simulink library "BrickPi"  (R2018b)
settings: Solver=VariableStepAuto  StartTime=0.0  StopTime=10.0  RelTol=1e-3
libraries: raspberrypilib x50, hdlsllib x27, xpcutilitieslib x18, $bdroot x1
(part 4 of 4)

== system BrickPi/Motor_Encoder/Get Encoder Value/Switch Case Action Subsystem/Subsystem/Motor_Offset ==
  note: Set offset value
  Offset : Inport  OutDataTypeStr=int32
  MotorPort : Inport  Port=2  OutDataTypeStr=uint8
  "Address " : Constant  OutDataTypeStr=uint8
  Bit Shift : hdlsllib/Logic and Bit Operations/Bit Shift  mode=Shift Right Logical  N=24
      settings: SourceProductName=HDL Coder  SourceProductBaseCode=HD
  Bit Shift1 : hdlsllib/Logic and Bit Operations/Bit Shift  mode=Shift Right Logical  N=16
      settings: SourceProductName=HDL Coder  SourceProductBaseCode=HD
  Bit Shift2 : hdlsllib/Logic and Bit Operations/Bit Shift  mode=Shift Right Logical  N=8
      settings: SourceProductName=HDL Coder  SourceProductBaseCode=HD
  Constant2 : Constant  OutDataTypeStr=uint8
  Constant3 : Constant  OutDataTypeStr=uint8
  Data Type Conversion{,1..3} (4 alike) : DataTypeConversion  OutDataTypeStr=uint8
  Mux2 : Mux  Inputs=7
  SPI Master Transfer2 : raspberrypilib/SPI Master Transfer  Priority=6  BoardProperty=Pi 3 Model B  SPIModule=uint32(0)  Mode=Master  BusSpeed=1000000  Pin=SPI0_CE1  FirstBitToTransfer=Most significant bit (MSB)  ClockMode=0  BlockFunction=Transfer  RegisterAddress=0  OutputDataType=int8  OutputDataLength=1
      settings: SourceProductName=Simulink Support Package for Raspberry Pi Hardware  SourceProductBaseCode=RASPPI
  SPI_MSG_ OFFSET_ENCODER : Constant  Value=29  OutMin=[1]  OutDataTypeStr=uint8
  Shift Arithmetic : ArithShift  BitShiftNumberSource=Input port  BitShiftNumber=8  BitShiftDirection=Left
      settings: InputPortMap=u0,p1
  Subtract : Sum  Inputs=+-
  Terminator : Terminator
  wires:
  Data Type Conversion/1 -> Mux2/4
  Data Type Conversion2/1 -> Mux2/6
  Offset/1 -> Bit Shift1/1, Bit Shift2/1, Data Type Conversion3/1, Bit Shift/1
  Constant2/1 -> Shift Arithmetic/1
  Bit Shift2/1 -> Data Type Conversion2/1
  Constant3/1 -> Subtract/2
  Bit Shift/1 -> Data Type Conversion/1
  Mux2/1 -> SPI Master Transfer2/1
  SPI Master Transfer2/1 -> Terminator/1
  Data Type Conversion3/1 -> Mux2/7
  Subtract/1 -> Shift Arithmetic/2
  MotorPort/1 -> Subtract/1
  Bit Shift1/1 -> Data Type Conversion1/1
  Data Type Conversion1/1 -> Mux2/5
  SPI_MSG_ OFFSET_ENCODER/1 -> Mux2/2
  "Address "/1 -> Mux2/1
  Shift Arithmetic/1 -> Mux2/3

== system BrickPi/Motor_Status/Get motor values/Switch Case Action Subsystem/Subsystem/Encoder ==
  note: Get motor encoder
  MotorPort : Inport
  0xA5 : Constant  Value=165
  "Address " : Constant  OutDataTypeStr=uint8
  Address3 : Constant  Value=[0 0 0 0 0 0 0 0]  OutDataTypeStr=uint8
  "Byte Packing " : xpcutilitieslib/Byte Packing   MaskPackedDataType=int32  MaskUnpackedDataTypes={'uint8', 'uint8', 'uint8', 'uint8'}  MaskAlignment=1
  Bytes[3-7] : Selector  IndexMode=Zero-based  InputPortWidth=10  IndexOptions=Index vector (dialog)  Indices=[3 4 5 6 7]  OutputSizes=1
  Demux : Demux  Outputs=5
  Mux2 : Mux  Inputs=3
  NAND : Logic  Operator=NAND  IconShape=distinctive  AllPortsSameDT=off  OutDataTypeStr=boolean
  SPI Master Transfer2 : raspberrypilib/SPI Master Transfer  Priority=6  BoardProperty=Pi 3 Model B  SPIModule=uint32(0)  Mode=Master  BusSpeed=1000000  Pin=SPI0_CE1  FirstBitToTransfer=Most significant bit (MSB)  ClockMode=0  BlockFunction=Transfer  RegisterAddress=0  OutputDataType=int8  OutputDataLength=1
      settings: SourceProductName=Simulink Support Package for Raspberry Pi Hardware  SourceProductBaseCode=RASPPI
  SPI_MSG_GET_ MOTOR_ENCODER offset : Constant  Value=29  OutDataTypeStr=uint8
  Sum : Sum  OutDataTypeStr=uint8
  Value : Outport
  Error : Outport  Port=2
  wires:
  Address3/1 -> Mux2/3
  NAND/1 -> Error/1
  Sum/1 -> Mux2/2
  Mux2/1 -> SPI Master Transfer2/1
  MotorPort/1 -> Sum/1
  Demux/5 -> "Byte Packing "/1
  "Address "/1 -> Mux2/1
  Demux/4 -> "Byte Packing "/2
  Demux/3 -> "Byte Packing "/3
  Demux/1 -> NAND/2
  0xA5/1 -> NAND/1
  Demux/2 -> "Byte Packing "/4
  "Byte Packing "/1 -> Value/1
  Bytes[3-7]/1 -> Demux/1
  SPI Master Transfer2/1 -> Bytes[3-7]/1
  SPI_MSG_GET_ MOTOR_ENCODER offset/1 -> Sum/2

== system BrickPi/Motor_Status/Get motor values/Switch Case Action Subsystem/Subsystem/Motor_Offset ==
  note: Set offset value
  Offset : Inport  OutDataTypeStr=int32
  MotorPort : Inport  Port=2  OutDataTypeStr=uint8
  "Address " : Constant  OutDataTypeStr=uint8
  Bit Shift : hdlsllib/Logic and Bit Operations/Bit Shift  mode=Shift Right Logical  N=24
      settings: SourceProductName=HDL Coder  SourceProductBaseCode=HD
  Bit Shift1 : hdlsllib/Logic and Bit Operations/Bit Shift  mode=Shift Right Logical  N=16
      settings: SourceProductName=HDL Coder  SourceProductBaseCode=HD
  Bit Shift2 : hdlsllib/Logic and Bit Operations/Bit Shift  mode=Shift Right Logical  N=8
      settings: SourceProductName=HDL Coder  SourceProductBaseCode=HD
  Constant2 : Constant  OutDataTypeStr=uint8
  Constant3 : Constant  OutDataTypeStr=uint8
  Data Type Conversion{,1..3} (4 alike) : DataTypeConversion  OutDataTypeStr=uint8
  Mux2 : Mux  Inputs=7
  SPI Master Transfer2 : raspberrypilib/SPI Master Transfer  Priority=6  BoardProperty=Pi 3 Model B  SPIModule=uint32(0)  Mode=Master  BusSpeed=1000000  Pin=SPI0_CE1  FirstBitToTransfer=Most significant bit (MSB)  ClockMode=0  BlockFunction=Transfer  RegisterAddress=0  OutputDataType=int8  OutputDataLength=1
      settings: SourceProductName=Simulink Support Package for Raspberry Pi Hardware  SourceProductBaseCode=RASPPI
  SPI_MSG_ OFFSET_ENCODER : Constant  Value=29  OutMin=[1]  OutDataTypeStr=uint8
  Shift Arithmetic : ArithShift  BitShiftNumberSource=Input port  BitShiftNumber=8  BitShiftDirection=Left
      settings: InputPortMap=u0,p1
  Subtract : Sum  Inputs=+-
  Terminator : Terminator
  wires:
  Data Type Conversion/1 -> Mux2/4
  Data Type Conversion2/1 -> Mux2/6
  Offset/1 -> Bit Shift1/1, Bit Shift2/1, Data Type Conversion3/1, Bit Shift/1
  Constant2/1 -> Shift Arithmetic/1
  Bit Shift2/1 -> Data Type Conversion2/1
  Constant3/1 -> Subtract/2
  Bit Shift/1 -> Data Type Conversion/1
  Mux2/1 -> SPI Master Transfer2/1
  SPI Master Transfer2/1 -> Terminator/1
  Data Type Conversion3/1 -> Mux2/7
  Subtract/1 -> Shift Arithmetic/2
  MotorPort/1 -> Subtract/1
  Bit Shift1/1 -> Data Type Conversion1/1
  Data Type Conversion1/1 -> Mux2/5
  SPI_MSG_ OFFSET_ENCODER/1 -> Mux2/2
  "Address "/1 -> Mux2/1
  Shift Arithmetic/1 -> Mux2/3
